simulink model "Zero_pole_Discrete"  (R2012b)
settings: Solver=ode45  StartTime=0.0  StopTime=10.0  RelTol=1e-3
settings Model: Creator=Faradars  LastModifiedBy=Faradars

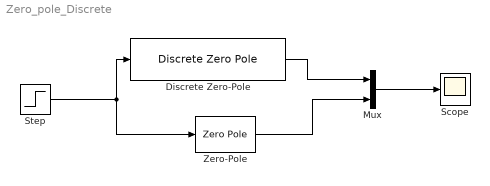
== system Zero_pole_Discrete ==
  Discrete Zero-Pole : DiscreteZeroPole  Zeros=[0.2023 0.6702 0.9048]  Poles=[0.8187 0.8187 0.7408 0.3679]  Gain=0.21493  SampleTime=0.1
  Mux : Mux  Inputs=2
  Scope : Scope
  Step : Step  SampleTime=0.1
  Zero-Pole : ZeroPole  Zeros=[-1 -4 -15]  Poles=[-2 -2 -3 -10]  Gain=2
  wires:
  Mux/1 -> Scope/1
  Step/1 -> Zero-Pole/1, Discrete Zero-Pole/1
  Zero-Pole/1 -> Mux/2
  Discrete Zero-Pole/1 -> Mux/1
